simulink model "PIDTest"  (R2013b)
settings: Solver=ode45  StartTime=0.0  StopTime=100  RelTol=1e-3
values from neighbouring files (symbols this model uses):
  C = C0    [Minimizer.m]    (also in parameters2.m = [1 0 0 0 0 0;0 0 1 0 0 0;0 0 0 0 1 0]; parameters3.m = [1 0 0 0 0 0;0 0 1 0 0 0;0 0 0 0 1 0])
  fw = 4    [parameters2.m]    (also in parameters3.m)
  I = 1/12*M*((2*rx1)^2 + (2*ry1)^2)    (= 7.46230507536)    [BoatController.m]    (also in boatDynamics.m; parameters2.m = 20; parameters3.m)
  k1m = 70    [parameters3.m]
  k1x = 50    [parameters3.m]
  k1y = 50    [parameters3.m]
  k2m = (4*k1m*I)^.5    (= 45.7104519897)    [parameters3.m]
  k2x = (4*k1x*M)^.5    (= 85.1907976251)    [parameters3.m]
  k2y = (4*k1y*M)^.5    (= 85.1907976251)    [parameters3.m]
  kr = 2    [parameters2.m]    (also in parameters3.m)
  M = 80*lbtokg    (= 36.28736)    [BoatController.m]    (also in parameters2.m = 10; parameters3.m)
libraries: simulink x3
settings Model: Creator=darsan13  LastModifiedBy=darsan13

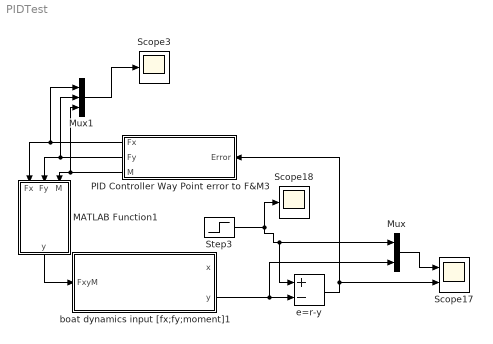
== system PIDTest ==
  MATLAB Function1 : MATLAB Function  TreatAsAtomicUnit=on
  Mux : Mux  Inputs=2
  Mux1 : Mux  Inputs=3
  PID Controller Way Point error to F&M3 : Subsystem
  Scope17 : Scope  NumInputPorts=2
      settings: YMin=-1~-5  YMax=1~5
  Scope18 : Scope
      settings: SaveName=ScopeData2
  Scope3 : Scope
      settings: SaveName=ScopeData5
  Step3 : Step  Before=[0;0;0]  After=[15;1;1]  SampleTime=0
  boat dynamics input [fx;fy;moment]1 : Subsystem  mask{M=M, I=I, fw=fw, kr=kr, C=C}
      mask prompts: M "Mass"; I "Inert"; fw "Water Friction"; kr "Rotational water Friction"; C "Output Matrix"
  e=r-y : Sum  Inputs=+-
  wires:
  Step3/1 -> e=r-y/1, Mux/1, Scope18/1
  e=r-y/1 -> PID Controller Way Point error to F&M3/1(Error), Scope17/2
  PID Controller Way Point error to F&M3/1(Fx) -> Mux1/1, MATLAB Function1/1(Fx)
  MATLAB Function1/1(y) -> boat dynamics input [fx;fy;moment]1/1(FxyM)
  PID Controller Way Point error to F&M3/2(Fy) -> Mux1/2, MATLAB Function1/2(Fy)
  PID Controller Way Point error to F&M3/3(M) -> Mux1/3, MATLAB Function1/3(M)
  boat dynamics input [fx;fy;moment]1/2(y) -> Mux/2, e=r-y/2
  Mux/1 -> Scope17/1
  Mux1/1 -> Scope3/1

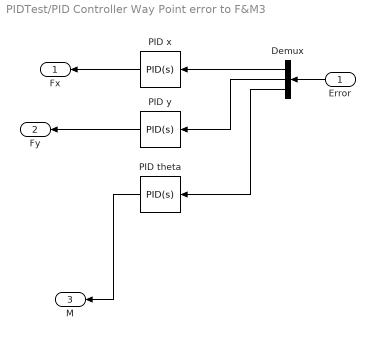
== system PIDTest/PID Controller Way Point error to F&M3 ==
  Error : Inport
  Demux : Demux  Outputs=3
  PID theta : simulink/Continuous/PID Controller  Controller=PID  TimeDomain=Continuous-time  SampleTime=1  IntegratorMethod=Forward Euler  FilterMethod=Forward Euler  Form=Parallel  P=k1m  I=0  D=k2m  N=3.646824066771  InitialConditionSource=internal  InitialConditionForIntegrator=0  InitialConditionForFilter=0  ExternalReset=none  LimitOutput=off  UpperSaturationLimit=inf  LowerSaturationLimit=-inf  LinearizeAsGain=off  AntiWindupMode=none  Kb=1  TrackingMode=off  Kt=1  PParamMin=[]  PParamMax=[]  IParamMin=[]  IParamMax=[]  DParamMin=[]  DParamMax=[]  NParamMin=[]  NParamMax=[]  KbParamMin=[]  KbParamMax=[]  KtParamMin=[]  KtParamMax=[]  POutMin=[]  POutMax=[]  IOutMin=[]  IOutMax=[]  DOutMin=[]  DOutMax=[]  NOutMin=[]  NOutMax=[]  KbOutMin=[]  KbOutMax=[]  KtOutMin=[]  KtOutMax=[]  IntegratorOutMin=[]  IntegratorOutMax=[]  FilterOutMin=[]  FilterOutMax=[]  SumOutMin=[]  SumOutMax=[]  SumI1OutMin=[]  SumI1OutMax=[]  SumI2OutMin=[]  SumI2OutMax=[]  SumI3OutMin=[]  SumI3OutMax=[]  SumDOutMin=[]  SumDOutMax=[]  SaturationOutMin=[]  SaturationOutMax=[]  IntegratorContinuousStateAttributes=''  IntegratorStateMustResolveToSignalObject=off  IntegratorRTWStateStorageClass=Auto  FilterContinuousStateAttributes=''  FilterStateMustResolveToSignalObject=off  FilterRTWStateStorageClass=Auto
  PID x : simulink/Continuous/PID Controller  Controller=PID  TimeDomain=Continuous-time  SampleTime=1  IntegratorMethod=Forward Euler  FilterMethod=Forward Euler  Form=Parallel  P=k1x  I=0  D=k2x  N=3.646824066771  InitialConditionSource=internal  InitialConditionForIntegrator=0  InitialConditionForFilter=0  ExternalReset=none  LimitOutput=off  UpperSaturationLimit=inf  LowerSaturationLimit=-inf  LinearizeAsGain=off  AntiWindupMode=none  Kb=1  TrackingMode=off  Kt=1  PParamMin=[]  PParamMax=[]  IParamMin=[]  IParamMax=[]  DParamMin=[]  DParamMax=[]  NParamMin=[]  NParamMax=[]  KbParamMin=[]  KbParamMax=[]  KtParamMin=[]  KtParamMax=[]  POutMin=[]  POutMax=[]  IOutMin=[]  IOutMax=[]  DOutMin=[]  DOutMax=[]  NOutMin=[]  NOutMax=[]  KbOutMin=[]  KbOutMax=[]  KtOutMin=[]  KtOutMax=[]  IntegratorOutMin=[]  IntegratorOutMax=[]  FilterOutMin=[]  FilterOutMax=[]  SumOutMin=[]  SumOutMax=[]  SumI1OutMin=[]  SumI1OutMax=[]  SumI2OutMin=[]  SumI2OutMax=[]  SumI3OutMin=[]  SumI3OutMax=[]  SumDOutMin=[]  SumDOutMax=[]  SaturationOutMin=[]  SaturationOutMax=[]  IntegratorContinuousStateAttributes=''  IntegratorStateMustResolveToSignalObject=off  IntegratorRTWStateStorageClass=Auto  FilterContinuousStateAttributes=''  FilterStateMustResolveToSignalObject=off  FilterRTWStateStorageClass=Auto
  PID y : simulink/Continuous/PID Controller  Controller=PID  TimeDomain=Continuous-time  SampleTime=1  IntegratorMethod=Forward Euler  FilterMethod=Forward Euler  Form=Parallel  P=k1y  I=0  D=k2y  N=4  InitialConditionSource=internal  InitialConditionForIntegrator=0  InitialConditionForFilter=0  ExternalReset=none  LimitOutput=off  UpperSaturationLimit=inf  LowerSaturationLimit=-inf  LinearizeAsGain=off  AntiWindupMode=none  Kb=1  TrackingMode=off  Kt=1  PParamMin=[]  PParamMax=[]  IParamMin=[]  IParamMax=[]  DParamMin=[]  DParamMax=[]  NParamMin=[]  NParamMax=[]  KbParamMin=[]  KbParamMax=[]  KtParamMin=[]  KtParamMax=[]  POutMin=[]  POutMax=[]  IOutMin=[]  IOutMax=[]  DOutMin=[]  DOutMax=[]  NOutMin=[]  NOutMax=[]  KbOutMin=[]  KbOutMax=[]  KtOutMin=[]  KtOutMax=[]  IntegratorOutMin=[]  IntegratorOutMax=[]  FilterOutMin=[]  FilterOutMax=[]  SumOutMin=[]  SumOutMax=[]  SumI1OutMin=[]  SumI1OutMax=[]  SumI2OutMin=[]  SumI2OutMax=[]  SumI3OutMin=[]  SumI3OutMax=[]  SumDOutMin=[]  SumDOutMax=[]  SaturationOutMin=[]  SaturationOutMax=[]  IntegratorContinuousStateAttributes=''  IntegratorStateMustResolveToSignalObject=off  IntegratorRTWStateStorageClass=Auto  FilterContinuousStateAttributes=''  FilterStateMustResolveToSignalObject=off  FilterRTWStateStorageClass=Auto
  Fx : Outport
  Fy : Outport  Port=2
  M : Outport  Port=3
  wires:
  Demux/1 -> PID x/1
  Demux/2 -> PID y/1
  Demux/3 -> PID theta/1
  Error/1 -> Demux/1
  PID y/1 -> Fy/1
  PID x/1 -> Fx/1
  PID theta/1 -> M/1

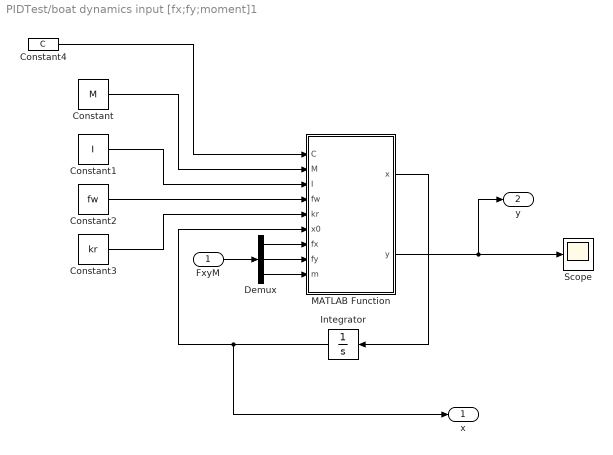
== system PIDTest/boat dynamics input [fx;fy;moment]1 ==
  FxyM : Inport
  Constant : Constant  Value=M
  Constant1 : Constant  Value=I
  Constant2 : Constant  Value=fw
  Constant3 : Constant  Value=kr
  Constant4 : Constant  Value=C
  Demux : Demux  Outputs=3
  Integrator : Integrator  InitialCondition=[0 0 0 0 0 0]
  MATLAB Function : MATLAB Function  TreatAsAtomicUnit=on
  Scope : Scope
  x : Outport
  y : Outport  Port=2
  wires:
  MATLAB Function/2(y) -> Scope/1, y/1
  Integrator/1 -> x/1, MATLAB Function/6(x0)
  Constant/1 -> MATLAB Function/2(M)
  Constant1/1 -> MATLAB Function/3(I)
  Constant2/1 -> MATLAB Function/4(fw)
  Constant3/1 -> MATLAB Function/5(kr)
  Constant4/1 -> MATLAB Function/1(C)
  MATLAB Function/1(x) -> Integrator/1
  FxyM/1 -> Demux/1
  Demux/1 -> MATLAB Function/7(fx)
  Demux/2 -> MATLAB Function/8(fy)
  Demux/3 -> MATLAB Function/9(m)

== matlab function PIDTest/MATLAB Function1 ==
  data: Fx input; y output; Fy input; M input
function y = fcn(Fx,Fy,M)
%#codegen

y = [Fx;Fy;M];

== matlab function PIDTest/boat dynamics input [fx;fy;moment]1/MATLAB Function ==
  data: C input; x output; M input; I input; fw input; kr input; x0 input; fx input; y output; fy input; m input
function [x,y] = systemstep(C,M,I,fw,kr,x0,fx,fy,m)

   % status vector y=[x;x_dot;y;_y_dot;theta;theta_dot]
   % forces u=[fx;fy;m]
   % contant parameters {mass; rotational inertia; friction coefficients }
   
   x1 = x0(2);
   x2 = fx/M - 0*x0(2)*fw;
   x3 = x0(4);
   x4 = fy/M - 0*x0(4)*fw;
   x5 = x0(6);
   x6 = m/I - 0*x0(6)*kr;

   x=[x1;x2;x3;x4;x5;x6];
   
   y = C*x0;
